simulink model "LUT_liver_pancreas_35"  (R2023b)
settings: Solver=FixedStepAuto  StartTime=0  StopTime=10.1  FixedStep=Timegap  RelTol=1e-3
model workspace (MAT data in the model file):
  T1_input = 1.34
(part 2 of 3)

== system LUT_liver_pancreas_35/If Action Subsystem6/If Action Subsystem1/If Action Subsystem6/If Action Subsystem3 ==
  In1 : Inport
  Action Port : ActionPort  ActionPortLabel=elseif( u1 >= 1.025)
  LUT 1.03RR : Lookup_n-D  NumberOfTableDimensions=1  BreakpointsForDimension1=[412.9882;555.7721;654.0253;752.1829;850.2431;948.2388;1046.193;1144.12;1242.028;1339.925;1437.812;1535.693;1633.569;1731.441;1829.31;1927.175;2025.037]  Table=[400;500;600;700;800;900;1000;1100;1200;1300;1400;1500;1600;1700;1800;1900;2000]  InternalRulePriority=Speed  RndMeth=Simplest
  Out1 : Outport
  wires:
  In1/1 -> LUT 1.03RR/1
  LUT 1.03RR/1 -> Out1/1

== system LUT_liver_pancreas_35/If Action Subsystem6/If Action Subsystem1/If Action Subsystem6/If Action Subsystem4 ==
  In1 : Inport
  Action Port : ActionPort  ActionPortLabel=elseif( u1 >= 1.035)
  LUT 1.04RR : Lookup_n-D  NumberOfTableDimensions=1  BreakpointsForDimension1=[412.8283;555.4024;653.5047;751.5005;849.3924;947.2154;1044.994;1142.743;1240.473;1338.189;1435.895;1533.595;1631.289;1728.979;1826.665;1924.348;2022.027]  Table=[400;500;600;700;800;900;1000;1100;1200;1300;1400;1500;1600;1700;1800;1900;2000]  InternalRulePriority=Speed  RndMeth=Simplest
  Out1 : Outport
  wires:
  In1/1 -> LUT 1.04RR/1
  LUT 1.04RR/1 -> Out1/1

== system LUT_liver_pancreas_35/If Action Subsystem6/If Action Subsystem1/If Action Subsystem6/If Action Subsystem5 ==
  In1 : Inport
  Action Port : ActionPort  ActionPortLabel=elseif( u1 >= 1.055)
  LUT 1.06RR : Lookup_n-D  NumberOfTableDimensions=1  BreakpointsForDimension1=[412.5162;554.689;652.5019;750.1865;847.7536;945.2432;1042.683;1140.089;1237.472;1334.84;1432.196;1529.544;1626.886;1724.223;1821.556;1918.886;2016.211]  Table=[400;500;600;700;800;900;1000;1100;1200;1300;1400;1500;1600;1700;1800;1900;2000]  InternalRulePriority=Speed  RndMeth=Simplest
  Out1 : Outport
  wires:
  In1/1 -> LUT 1.06RR/1
  LUT 1.06RR/1 -> Out1/1

== system LUT_liver_pancreas_35/If Action Subsystem6/If Action Subsystem1/If Action Subsystem6/If Action Subsystem6 ==
  In1 : Inport
  Action Port : ActionPort  ActionPortLabel=elseif( u1 >= 1.045)
  LUT 1.05RR : Lookup_n-D  NumberOfTableDimensions=1  BreakpointsForDimension1=[412.671;555.0414;652.997;750.8352;848.5627;946.2171;1043.824;1141.4;1238.955;1336.494;1434.024;1531.546;1629.062;1726.574;1824.081;1921.586;2019.086]  Table=[400;500;600;700;800;900;1000;1100;1200;1300;1400;1500;1600;1700;1800;1900;2000]  InternalRulePriority=Speed  RndMeth=Simplest
  Out1 : Outport
  wires:
  In1/1 -> LUT 1.05RR/1
  LUT 1.05RR/1 -> Out1/1

== system LUT_liver_pancreas_35/If Action Subsystem6/If Action Subsystem1/If Action Subsystem6/If Action Subsystem7 ==
  In1 : Inport
  Action Port : ActionPort  ActionPortLabel=elseif( u1 >= 1.065)
  LUT 1.07RR : Lookup_n-D  NumberOfTableDimensions=1  BreakpointsForDimension1=[412.364;554.3449;652.019;749.5538;846.9643;944.293;1041.568;1138.808;1236.024;1333.224;1430.411;1527.589;1624.76;1721.926;1819.088;1916.246;2013.4]  Table=[400;500;600;700;800;900;1000;1100;1200;1300;1400;1500;1600;1700;1800;1900;2000]  InternalRulePriority=Speed  RndMeth=Simplest
  Out1 : Outport
  wires:
  In1/1 -> LUT 1.07RR/1
  LUT 1.07RR/1 -> Out1/1

== system LUT_liver_pancreas_35/If Action Subsystem6/If Action Subsystem1/If Action Subsystem6/If Action Subsystem8 ==
  In1 : Inport
  Action Port : ActionPort  ActionPortLabel=elseif(u1 >= 1.075)
  LUT 1.08RR : Lookup_n-D  NumberOfTableDimensions=1  BreakpointsForDimension1=[412.2141;554.0089;651.5479;748.9366;846.1942;943.3656;1040.481;1137.558;1234.611;1331.645;1428.666;1525.678;1622.682;1719.681;1816.676;1913.666;2010.652]  Table=[400;500;600;700;800;900;1000;1100;1200;1300;1400;1500;1600;1700;1800;1900;2000]  InternalRulePriority=Speed  RndMeth=Simplest
  Out1 : Outport
  wires:
  In1/1 -> LUT 1.08RR/1
  LUT 1.08RR/1 -> Out1/1

== system LUT_liver_pancreas_35/If Action Subsystem6/If Action Subsystem1/If Action Subsystem6/If Action Subsystem9 ==
  In1 : Inport
  Action Port : ActionPort  ActionPortLabel=if(u1 >= 1.085)
  LUT 1.09RR : Lookup_n-D  NumberOfTableDimensions=1  BreakpointsForDimension1=[412.0667;553.6807;651.0883;748.3345;845.4429;942.4605;1039.419;1136.338;1233.23;1330.102;1426.961;1523.81;1620.651;1717.486;1814.317;1911.142;2007.964]  Table=[400;500;600;700;800;900;1000;1100;1200;1300;1400;1500;1600;1700;1800;1900;2000]  InternalRulePriority=Speed  RndMeth=Simplest
  Out1 : Outport
  wires:
  In1/1 -> LUT 1.09RR/1
  LUT 1.09RR/1 -> Out1/1

== system LUT_liver_pancreas_35/If Action Subsystem6/If Action Subsystem1/If Action Subsystem7/If Action Subsystem1 ==
  In1 : Inport
  Action Port : ActionPort  ActionPortLabel=elseif( u1 >= 1.215)
  LUT 1.22RR : Lookup_n-D  NumberOfTableDimensions=1  BreakpointsForDimension1=[410.344;550.0322;646.0176;741.6977;837.1488;932.4494;1027.65;1122.782;1217.866;1312.916;1407.94;1502.945;1597.935;1692.914;1787.883;1882.845;1977.801]  Table=[400;500;600;700;800;900;1000;1100;1200;1300;1400;1500;1600;1700;1800;1900;2000]  InternalRulePriority=Speed  RndMeth=Simplest
  Out1 : Outport
  wires:
  In1/1 -> LUT 1.22RR/1
  LUT 1.22RR/1 -> Out1/1

== system LUT_liver_pancreas_35/If Action Subsystem6/If Action Subsystem1/If Action Subsystem7/If Action Subsystem10 ==
  In1 : Inport
  Action Port : ActionPort  ActionPortLabel=elseif( u1 >= 1.205)
  LUT 1.21RR : Lookup_n-D  NumberOfTableDimensions=1  BreakpointsForDimension1=[410.4648;550.2769;646.3551;742.1389;837.701;933.1173;1028.437;1123.69;1218.897;1314.071;1409.22;1504.351;1599.467;1694.573;1789.67;1884.759;1979.843]  Table=[400;500;600;700;800;900;1000;1100;1200;1300;1400;1500;1600;1700;1800;1900;2000]  InternalRulePriority=Speed  RndMeth=Simplest
  Out1 : Outport
  wires:
  In1/1 -> LUT 1.21RR/1
  LUT 1.21RR/1 -> Out1/1

== system LUT_liver_pancreas_35/If Action Subsystem6/If Action Subsystem1/If Action Subsystem7/If Action Subsystem2 ==
  In1 : Inport
  Action Port : ActionPort  ActionPortLabel=else
  LUT 1.20RR : Lookup_n-D  NumberOfTableDimensions=1  BreakpointsForDimension1=[410.5875;550.527;646.7004;742.5906;838.2661;933.8005;1029.241;1124.618;1219.951;1315.251;1410.528;1505.787;1601.032;1696.267;1791.493;1886.713;1981.926]  Table=[400;500;600;700;800;900;1000;1100;1200;1300;1400;1500;1600;1700;1800;1900;2000]  InternalRulePriority=Speed  RndMeth=Simplest
  Out1 : Outport
  wires:
  In1/1 -> LUT 1.20RR/1
  LUT 1.20RR/1 -> Out1/1

== system LUT_liver_pancreas_35/If Action Subsystem6/If Action Subsystem1/If Action Subsystem7/If Action Subsystem3 ==
  In1 : Inport
  Action Port : ActionPort  ActionPortLabel=elseif( u1 >= 1.225)
  LUT 1.23RR : Lookup_n-D  NumberOfTableDimensions=1  BreakpointsForDimension1=[410.2248;549.7928;645.6879;741.2665;836.6092;931.7964;1026.88;1121.894;1216.857;1311.785;1406.686;1501.568;1596.434;1691.288;1786.133;1880.969;1975.8]  Table=[400;500;600;700;800;900;1000;1100;1200;1300;1400;1500;1600;1700;1800;1900;2000]  InternalRulePriority=Speed  RndMeth=Simplest
  Out1 : Outport
  wires:
  In1/1 -> LUT 1.23RR/1
  LUT 1.23RR/1 -> Out1/1

== system LUT_liver_pancreas_35/If Action Subsystem6/If Action Subsystem1/If Action Subsystem7/If Action Subsystem4 ==
  In1 : Inport
  Action Port : ActionPort  ActionPortLabel=elseif( u1 >= 1.235)
  LUT 1.24RR : Lookup_n-D  NumberOfTableDimensions=1  BreakpointsForDimension1=[410.1074;549.5585;645.3656;740.8452;836.0817;931.158;1026.128;1121.024;1215.87;1310.678;1405.459;1500.219;1594.963;1689.695;1784.417;1879.131;1973.838]  Table=[400;500;600;700;800;900;1000;1100;1200;1300;1400;1500;1600;1700;1800;1900;2000]  InternalRulePriority=Speed  RndMeth=Simplest
  Out1 : Outport
  wires:
  In1/1 -> LUT 1.24RR/1
  LUT 1.24RR/1 -> Out1/1

== system LUT_liver_pancreas_35/If Action Subsystem6/If Action Subsystem1/If Action Subsystem7/If Action Subsystem5 ==
  In1 : Inport
  Action Port : ActionPort  ActionPortLabel=elseif( u1 >= 1.255)
  LUT 1.26RR : Lookup_n-D  NumberOfTableDimensions=1  BreakpointsForDimension1=[409.8775;549.1047;644.7426;740.031;835.062;929.9232;1024.671;1119.341;1213.957;1308.533;1403.079;1497.603;1592.111;1686.605;1781.088;1875.562;1970.03]  Table=[400;500;600;700;800;900;1000;1100;1200;1300;1400;1500;1600;1700;1800;1900;2000]  InternalRulePriority=Speed  RndMeth=Simplest
  Out1 : Outport
  wires:
  In1/1 -> LUT 1.26RR/1
  LUT 1.26RR/1 -> Out1/1

== system LUT_liver_pancreas_35/If Action Subsystem6/If Action Subsystem1/If Action Subsystem7/If Action Subsystem6 ==
  In1 : Inport
  Action Port : ActionPort  ActionPortLabel=elseif( u1 >= 1.245)
  LUT 1.25RR : Lookup_n-D  NumberOfTableDimensions=1  BreakpointsForDimension1=[409.9916;549.3292;645.0505;740.4334;835.566;930.5337;1025.391;1120.174;1214.903;1309.594;1404.257;1498.898;1593.522;1688.134;1782.736;1877.329;1971.915]  Table=[400;500;600;700;800;900;1000;1100;1200;1300;1400;1500;1600;1700;1800;1900;2000]  InternalRulePriority=Speed  RndMeth=Simplest
  Out1 : Outport
  wires:
  In1/1 -> LUT 1.25RR/1
  LUT 1.25RR/1 -> Out1/1

== system LUT_liver_pancreas_35/If Action Subsystem6/If Action Subsystem1/If Action Subsystem7/If Action Subsystem7 ==
  In1 : Inport
  Action Port : ActionPort  ActionPortLabel=elseif( u1 >= 1.265)
  LUT 1.27RR : Lookup_n-D  NumberOfTableDimensions=1  BreakpointsForDimension1=[409.765;548.8849;644.4415;739.6376;834.5691;929.3261;1023.966;1118.527;1213.03;1307.493;1401.926;1496.335;1590.727;1685.105;1779.472;1873.83;1968.181]  Table=[400;500;600;700;800;900;1000;1100;1200;1300;1400;1500;1600;1700;1800;1900;2000]  InternalRulePriority=Speed  RndMeth=Simplest
  Out1 : Outport
  wires:
  In1/1 -> LUT 1.27RR/1
  LUT 1.27RR/1 -> Out1/1

== system LUT_liver_pancreas_35/If Action Subsystem6/If Action Subsystem1/If Action Subsystem7/If Action Subsystem8 ==
  In1 : Inport
  Action Port : ActionPort  ActionPortLabel=elseif(u1 >= 1.275)
  LUT 1.28RR : Lookup_n-D  NumberOfTableDimensions=1  BreakpointsForDimension1=[409.654;548.6697;644.1471;739.2531;834.0873;928.7421;1023.277;1117.729;1212.123;1306.475;1400.796;1495.093;1589.371;1683.635;1777.888;1872.132;1966.368]  Table=[400;500;600;700;800;900;1000;1100;1200;1300;1400;1500;1600;1700;1800;1900;2000]  InternalRulePriority=Speed  RndMeth=Simplest
  Out1 : Outport
  wires:
  In1/1 -> LUT 1.28RR/1
  LUT 1.28RR/1 -> Out1/1

== system LUT_liver_pancreas_35/If Action Subsystem6/If Action Subsystem1/If Action Subsystem7/If Action Subsystem9 ==
  In1 : Inport
  Action Port : ActionPort  ActionPortLabel=if(u1 >= 1.285)
  LUT 1.29RR : Lookup_n-D  NumberOfTableDimensions=1  BreakpointsForDimension1=[409.5446;548.459;643.8592;738.8772;833.6161;928.1708;1022.602;1116.949;1211.235;1305.478;1399.689;1493.875;1588.042;1682.195;1776.335;1870.466;1964.589]  Table=[400;500;600;700;800;900;1000;1100;1200;1300;1400;1500;1600;1700;1800;1900;2000]  InternalRulePriority=Speed  RndMeth=Simplest
  Out1 : Outport
  wires:
  In1/1 -> LUT 1.29RR/1
  LUT 1.29RR/1 -> Out1/1

== system LUT_liver_pancreas_35/If Action Subsystem6/If Action Subsystem1/If Action Subsystem8/If Action Subsystem1 ==
  In1 : Inport
  Action Port : ActionPort  ActionPortLabel=elseif( u1 >= 1.315)
  LUT 1.32RR : Lookup_n-D  NumberOfTableDimensions=1  BreakpointsForDimension1=[409.2254;547.8525;643.0331;737.7988;832.2639;926.5301;1020.663;1114.703;1208.679;1302.606;1396.499;1490.364;1584.209;1678.038;1771.853;1865.658;1959.455]  Table=[400;500;600;700;800;900;1000;1100;1200;1300;1400;1500;1600;1700;1800;1900;2000]  InternalRulePriority=Speed  RndMeth=Simplest
  Out1 : Outport
  wires:
  In1/1 -> LUT 1.32RR/1
  LUT 1.32RR/1 -> Out1/1

== system LUT_liver_pancreas_35/If Action Subsystem6/If Action Subsystem1/If Action Subsystem8/If Action Subsystem10 ==
  In1 : Inport
  Action Port : ActionPort  ActionPortLabel=elseif( u1 >= 1.305)
  LUT 1.31RR : Lookup_n-D  NumberOfTableDimensions=1  BreakpointsForDimension1=[409.3303;548.0505;643.3024;738.1503;832.7047;927.0651;1021.295;1115.436;1209.513;1303.544;1397.541;1491.511;1585.462;1679.396;1773.318;1867.23;1961.134]  Table=[400;500;600;700;800;900;1000;1100;1200;1300;1400;1500;1600;1700;1800;1900;2000]  InternalRulePriority=Speed  RndMeth=Simplest
  Out1 : Outport
  wires:
  In1/1 -> LUT 1.31RR/1
  LUT 1.31RR/1 -> Out1/1

== system LUT_liver_pancreas_35/If Action Subsystem6/If Action Subsystem1/If Action Subsystem8/If Action Subsystem2 ==
  In1 : Inport
  Action Port : ActionPort  ActionPortLabel=else
  LUT 1.30RR : Lookup_n-D  NumberOfTableDimensions=1  BreakpointsForDimension1=[409.4368;548.2526;643.5777;738.5096;833.1553;927.6119;1021.942;1116.184;1210.365;1304.501;1398.604;1492.681;1586.739;1680.782;1774.812;1868.833;1962.845]  Table=[400;500;600;700;800;900;1000;1100;1200;1300;1400;1500;1600;1700;1800;1900;2000]  InternalRulePriority=Speed  RndMeth=Simplest
  Out1 : Outport
  wires:
  In1/1 -> LUT 1.30RR/1
  LUT 1.30RR/1 -> Out1/1

== system LUT_liver_pancreas_35/If Action Subsystem6/If Action Subsystem1/If Action Subsystem8/If Action Subsystem3 ==
  In1 : Inport
  Action Port : ActionPort  ActionPortLabel=elseif( u1 >= 1.325)
  LUT 1.33RR : Lookup_n-D  NumberOfTableDimensions=1  BreakpointsForDimension1=[409.1218;547.6585;642.7698;737.4552;831.8328;926.0066;1020.044;1113.986;1207.861;1301.687;1395.478;1489.24;1582.981;1676.705;1770.416;1864.116;1957.807]  Table=[400;500;600;700;800;900;1000;1100;1200;1300;1400;1500;1600;1700;1800;1900;2000]  InternalRulePriority=Speed  RndMeth=Simplest
  Out1 : Outport
  wires:
  In1/1 -> LUT 1.33RR/1
  LUT 1.33RR/1 -> Out1/1

== system LUT_liver_pancreas_35/If Action Subsystem6/If Action Subsystem1/If Action Subsystem8/If Action Subsystem4 ==
  In1 : Inport
  Action Port : ActionPort  ActionPortLabel=elseif( u1 >= 1.335)
  LUT 1.34RR : Lookup_n-D  NumberOfTableDimensions=1  BreakpointsForDimension1=[409.0197;547.4685;642.5121;737.1191;831.4111;925.4944;1019.437;1113.283;1207.06;1300.787;1394.476;1488.137;1581.776;1675.398;1769.006;1862.603;1956.19]  Table=[400;500;600;700;800;900;1000;1100;1200;1300;1400;1500;1600;1700;1800;1900;2000]  InternalRulePriority=Speed  RndMeth=Simplest
  Out1 : Outport
  wires:
  In1/1 -> LUT 1.34RR/1
  LUT 1.34RR/1 -> Out1/1

== system LUT_liver_pancreas_35/If Action Subsystem6/If Action Subsystem1/If Action Subsystem8/If Action Subsystem5 ==
  In1 : Inport
  Action Port : ActionPort  ActionPortLabel=elseif( u1 >= 1.355)
  LUT 1.36RR : Lookup_n-D  NumberOfTableDimensions=1  BreakpointsForDimension1=[408.8194;547.0998;642.0134;736.4689;830.595;924.5024;1018.263;1111.921;1205.507;1299.039;1392.533;1485.996;1579.436;1672.858;1766.265;1859.66;1953.046]  Table=[400;500;600;700;800;900;1000;1100;1200;1300;1400;1500;1600;1700;1800;1900;2000]  InternalRulePriority=Speed  RndMeth=Simplest
  Out1 : Outport
  wires:
  In1/1 -> LUT 1.36RR/1
  LUT 1.36RR/1 -> Out1/1

== system LUT_liver_pancreas_35/If Action Subsystem6/If Action Subsystem1/If Action Subsystem8/If Action Subsystem6 ==
  In1 : Inport
  Action Port : ActionPort  ActionPortLabel=elseif( u1 >= 1.345)
  LUT 1.35RR : Lookup_n-D  NumberOfTableDimensions=1  BreakpointsForDimension1=[408.9189;547.2823;642.26;736.7904;830.9986;924.9931;1018.844;1112.595;1206.276;1299.904;1393.495;1487.056;1580.595;1674.116;1767.623;1861.118;1954.603]  Table=[400;500;600;700;800;900;1000;1100;1200;1300;1400;1500;1600;1700;1800;1900;2000]  InternalRulePriority=Speed  RndMeth=Simplest
  Out1 : Outport
  wires:
  In1/1 -> LUT 1.35RR/1
  LUT 1.35RR/1 -> Out1/1

== system LUT_liver_pancreas_35/If Action Subsystem6/If Action Subsystem1/If Action Subsystem8/If Action Subsystem7 ==
  In1 : Inport
  Action Port : ActionPort  ActionPortLabel=elseif( u1 >= 1.365)
  LUT 1.37RR : Lookup_n-D  NumberOfTableDimensions=1  BreakpointsForDimension1=[408.7213;546.921;641.7721;736.1544;830.2001;924.0222;1017.694;1111.261;1204.753;1298.192;1391.589;1484.956;1578.299;1671.624;1764.933;1858.23;1951.517]  Table=[400;500;600;700;800;900;1000;1100;1200;1300;1400;1500;1600;1700;1800;1900;2000]  InternalRulePriority=Speed  RndMeth=Simplest
  Out1 : Outport
  wires:
  In1/1 -> LUT 1.37RR/1
  LUT 1.37RR/1 -> Out1/1

== system LUT_liver_pancreas_35/If Action Subsystem6/If Action Subsystem1/If Action Subsystem8/If Action Subsystem8 ==
  In1 : Inport
  Action Port : ActionPort  ActionPortLabel=elseif(u1 >= 1.375)
  LUT 1.38RR : Lookup_n-D  NumberOfTableDimensions=1  BreakpointsForDimension1=[408.6244;546.7457;641.5359;735.8468;829.8137;923.5522;1017.136;1110.614;1204.015;1297.36;1390.664;1483.937;1577.184;1670.413;1763.625;1856.826;1950.016]  Table=[400;500;600;700;800;900;1000;1100;1200;1300;1400;1500;1600;1700;1800;1900;2000]  InternalRulePriority=Speed  RndMeth=Simplest
  Out1 : Outport
  wires:
  In1/1 -> LUT 1.38RR/1
  LUT 1.38RR/1 -> Out1/1

== system LUT_liver_pancreas_35/If Action Subsystem6/If Action Subsystem1/If Action Subsystem8/If Action Subsystem9 ==
  In1 : Inport
  Action Port : ActionPort  ActionPortLabel=if(u1 >= 1.385)
  LUT 1.39RR : Lookup_n-D  NumberOfTableDimensions=1  BreakpointsForDimension1=[408.5288;546.5738;641.3049;735.5459;829.4357;923.0921;1016.591;1109.98;1203.291;1296.545;1389.757;1482.936;1576.09;1669.224;1762.342;1855.447;1948.542]  Table=[400;500;600;700;800;900;1000;1100;1200;1300;1400;1500;1600;1700;1800;1900;2000]  InternalRulePriority=Speed  RndMeth=Simplest
  Out1 : Outport
  wires:
  In1/1 -> LUT 1.39RR/1
  LUT 1.39RR/1 -> Out1/1

== system LUT_liver_pancreas_35/If Action Subsystem6/If Action Subsystem1/If Action Subsystem9/If Action Subsystem1 ==
  In1 : Inport
  Action Port : ActionPort  ActionPortLabel=elseif( u1 >= 1.415)
  LUT 1.42RR : Lookup_n-D  NumberOfTableDimensions=1  BreakpointsForDimension1=[408.2493167;546.0782587;640.6407138;734.6814994;828.3494623;921.7690503;1015.020415;1108.154745;1201.205449;1294.194915;1387.138542;1480.047175;1572.92862;1665.788602;1758.631391;1851.460216;1944.277551]  Table=[400;500;600;700;800;900;1000;1100;1200;1300;1400;1500;1600;1700;1800;1900;2000]  InternalRulePriority=Speed  RndMeth=Simplest
  Out1 : Outport
  wires:
  In1/1 -> LUT 1.42RR/1
  LUT 1.42RR/1 -> Out1/1

== system LUT_liver_pancreas_35/If Action Subsystem6/If Action Subsystem1/If Action Subsystem9/If Action Subsystem10 ==
  In1 : Inport
  Action Port : ActionPort  ActionPortLabel=elseif( u1 >= 1.405)
  LUT 1.41RR : Lookup_n-D  NumberOfTableDimensions=1  BreakpointsForDimension1=[408.3412832;546.2402113;640.8573639;734.9633581;828.7037439;922.2007473;1015.533048;1108.750853;1201.886902;1294.96312;1387.994576;1480.99188;1573.962659;1666.912507;1759.845592;1852.765065;1945.673336]  Table=[400;500;600;700;800;900;1000;1100;1200;1300;1400;1500;1600;1700;1800;1900;2000]  InternalRulePriority=Speed  RndMeth=Simplest
  Out1 : Outport
  wires:
  In1/1 -> LUT 1.41RR/1
  LUT 1.41RR/1 -> Out1/1

== system LUT_liver_pancreas_35/If Action Subsystem6/If Action Subsystem1/If Action Subsystem9/If Action Subsystem2 ==
  In1 : Inport
  Action Port : ActionPort  ActionPortLabel=else
  LUT 1.40RR : Lookup_n-D  NumberOfTableDimensions=1  BreakpointsForDimension1=[408.4344;546.4054;641.0787;735.2514;829.0658;922.6417;1016.056;1109.359;1202.582;1295.747;1388.867;1481.955;1575.016;1668.057;1761.082;1854.094;1947.095]  Table=[400;500;600;700;800;900;1000;1100;1200;1300;1400;1500;1600;1700;1800;1900;2000]  InternalRulePriority=Speed  RndMeth=Simplest
  Out1 : Outport
  wires:
  In1/1 -> LUT 1.40RR/1
  LUT 1.40RR/1 -> Out1/1

== system LUT_liver_pancreas_35/If Action Subsystem6/If Action Subsystem1/If Action Subsystem9/If Action Subsystem3 ==
  In1 : Inport
  Action Port : ActionPort  ActionPortLabel=elseif( u1 >= 1.425)
  LUT 1.43RR : Lookup_n-D  NumberOfTableDimensions=1  BreakpointsForDimension1=[408.1585;545.9194;640.4286;734.4057;828.0027;921.3464;1014.518;1107.571;1200.537;1293.442;1386.299;1479.12;1571.914;1664.685;1757.439;1850.179;1942.907]  Table=[400;500;600;700;800;900;1000;1100;1200;1300;1400;1500;1600;1700;1800;1900;2000]  InternalRulePriority=Speed  RndMeth=Simplest
  Out1 : Outport
  wires:
  In1/1 -> LUT 1.43RR/1
  LUT 1.43RR/1 -> Out1/1

== system LUT_liver_pancreas_35/If Action Subsystem6/If Action Subsystem1/If Action Subsystem9/If Action Subsystem4 ==
  In1 : Inport
  Action Port : ActionPort  ActionPortLabel=elseif( u1 >= 1.435)
  LUT 1.44RR : Lookup_n-D  NumberOfTableDimensions=1  BreakpointsForDimension1=[408.0689;545.7637;640.221;734.1358;827.6634;920.9325;1014.026;1106.998;1199.882;1292.703;1385.475;1478.211;1570.918;1663.602;1756.269;1848.92;1941.56]  Table=[400;500;600;700;800;900;1000;1100;1200;1300;1400;1500;1600;1700;1800;1900;2000]  InternalRulePriority=Speed  RndMeth=Simplest
  Out1 : Outport
  wires:
  In1/1 -> LUT 1.44RR/1
  LUT 1.44RR/1 -> Out1/1

== system LUT_liver_pancreas_35/If Action Subsystem6/If Action Subsystem1/If Action Subsystem9/If Action Subsystem5 ==
  In1 : Inport
  Action Port : ActionPort  ActionPortLabel=elseif( u1 >= 1.455)
  LUT 1.46RR : Lookup_n-D  NumberOfTableDimensions=1  BreakpointsForDimension1=[407.8929;545.4611;639.8188;733.6133;827.0061;920.1305;1013.073;1105.887;1198.611;1291.267;1383.874;1476.442;1568.98;1661.494;1753.99;1846.47;1938.937]  Table=[400;500;600;700;800;900;1000;1100;1200;1300;1400;1500;1600;1700;1800;1900;2000]  InternalRulePriority=Speed  RndMeth=Simplest
  Out1 : Outport
  wires:
  In1/1 -> LUT 1.46RR/1
  LUT 1.46RR/1 -> Out1/1

== system LUT_liver_pancreas_35/If Action Subsystem6/If Action Subsystem1/If Action Subsystem9/If Action Subsystem6 ==
  In1 : Inport
  Action Port : ActionPort  ActionPortLabel=elseif( u1 >= 1.445)
  LUT 1.45RR : Lookup_n-D  NumberOfTableDimensions=1  BreakpointsForDimension1=[407.9803;545.6109;640.0178;733.8717;827.3312;920.5273;1013.545;1106.437;1199.24;1291.978;1384.667;1477.318;1569.94;1662.539;1755.119;1847.684;1940.237]  Table=[400;500;600;700;800;900;1000;1100;1200;1300;1400;1500;1600;1700;1800;1900;2000]  InternalRulePriority=Speed  RndMeth=Simplest
  Out1 : Outport
  wires:
  In1/1 -> LUT 1.45RR/1
  LUT 1.45RR/1 -> Out1/1

== system LUT_liver_pancreas_35/If Action Subsystem6/If Action Subsystem1/If Action Subsystem9/If Action Subsystem7 ==
  In1 : Inport
  Action Port : ActionPort  ActionPortLabel=elseif( u1 >= 1.465)
  LUT 1.47RR : Lookup_n-D  NumberOfTableDimensions=1  BreakpointsForDimension1=[407.8066;545.3141;639.624;733.3604;826.6879;919.7419;1012.61;1105.348;1197.993;1290.57;1383.096;1475.582;1568.037;1660.469;1752.881;1845.277;1937.66]  Table=[400;500;600;700;800;900;1000;1100;1200;1300;1400;1500;1600;1700;1800;1900;2000]  InternalRulePriority=Speed  RndMeth=Simplest
  Out1 : Outport
  wires:
  In1/1 -> LUT 1.47RR/1
  LUT 1.47RR/1 -> Out1/1

== system LUT_liver_pancreas_35/If Action Subsystem6/If Action Subsystem1/If Action Subsystem9/If Action Subsystem8 ==
  In1 : Inport
  Action Port : ActionPort  ActionPortLabel=elseif(u1 >= 1.475)
  LUT 1.48RR : Lookup_n-D  NumberOfTableDimensions=1  BreakpointsForDimension1=[407.7213;545.1698;639.4333;733.1128;826.3764;919.3614;1012.157;1104.82;1197.388;1289.886;1382.332;1474.738;1567.112;1659.462;1751.792;1844.105;1936.406]  Table=[400;500;600;700;800;900;1000;1100;1200;1300;1400;1500;1600;1700;1800;1900;2000]  InternalRulePriority=Speed  RndMeth=Simplest
  Out1 : Outport
  wires:
  In1/1 -> LUT 1.48RR/1
  LUT 1.48RR/1 -> Out1/1

== system LUT_liver_pancreas_35/If Action Subsystem6/If Action Subsystem1/If Action Subsystem9/If Action Subsystem9 ==
  In1 : Inport
  Action Port : ActionPort  ActionPortLabel=if(u1 >= 1.485)
  LUT 1.49RR : Lookup_n-D  NumberOfTableDimensions=1  BreakpointsForDimension1=[407.637;545.0283;639.2465;732.8705;826.0714;918.9888;1011.713;1104.302;1196.794;1289.215;1381.583;1473.909;1566.203;1658.473;1750.721;1842.954;1935.173]  Table=[400;500;600;700;800;900;1000;1100;1200;1300;1400;1500;1600;1700;1800;1900;2000]  InternalRulePriority=Speed  RndMeth=Simplest
  Out1 : Outport
  wires:
  In1/1 -> LUT 1.49RR/1
  LUT 1.49RR/1 -> Out1/1

== system LUT_liver_pancreas_35/If Action Subsystem6/If Action Subsystem2/If Action Subsystem5/If Action Subsystem1 ==
  In1 : Inport
  Action Port : ActionPort  ActionPortLabel=elseif( u1 >= 1.615)
  LUT 1.62RR : Lookup_n-D  NumberOfTableDimensions=1  BreakpointsForDimension1=[406.6287;543.4093;637.1404;730.1493;822.6427;914.7867;1006.69;1098.424;1190.035;1281.556;1373.008;1464.407;1555.765;1647.09;1738.389;1829.666;1920.925]  Table=[400;500;600;700;800;900;1000;1100;1200;1300;1400;1500;1600;1700;1800;1900;2000]  InternalRulePriority=Speed  RndMeth=Simplest
  Out1 : Outport
  wires:
  In1/1 -> LUT 1.62RR/1
  LUT 1.62RR/1 -> Out1/1

== system LUT_liver_pancreas_35/If Action Subsystem6/If Action Subsystem2/If Action Subsystem5/If Action Subsystem10 ==
  In1 : Inport
  Action Port : ActionPort  ActionPortLabel=elseif( u1>= 1.605)
  LUT 1.61RR : Lookup_n-D  NumberOfTableDimensions=1  BreakpointsForDimension1=[406.701;543.5206;637.2832;730.333;822.8743;915.0714;1007.032;1098.825;1190.498;1282.081;1373.597;1465.061;1556.485;1647.877;1739.242;1830.587;1921.914]  Table=[400;500;600;700;800;900;1000;1100;1200;1300;1400;1500;1600;1700;1800;1900;2000]  InternalRulePriority=Speed  RndMeth=Simplest
  Out1 : Outport
  wires:
  In1/1 -> LUT 1.61RR/1
  LUT 1.61RR/1 -> Out1/1

== system LUT_liver_pancreas_35/If Action Subsystem6/If Action Subsystem2/If Action Subsystem5/If Action Subsystem2 ==
  In1 : Inport
  Action Port : ActionPort  ActionPortLabel=else
  LUT 1.60RR : Lookup_n-D  NumberOfTableDimensions=1  BreakpointsForDimension1=[406.7741;543.634;637.4289;730.5206;823.1109;915.362;1007.38;1099.234;1190.969;1282.616;1374.197;1465.728;1557.218;1648.677;1740.111;1831.523;1922.919]  Table=[400;500;600;700;800;900;1000;1100;1200;1300;1400;1500;1600;1700;1800;1900;2000]  InternalRulePriority=Speed  RndMeth=Simplest
  Out1 : Outport
  wires:
  In1/1 -> LUT 1.60RR/1
  LUT 1.60RR/1 -> Out1/1

== system LUT_liver_pancreas_35/If Action Subsystem6/If Action Subsystem2/If Action Subsystem5/If Action Subsystem3 ==
  In1 : Inport
  Action Port : ActionPort  ActionPortLabel=elseif( u1 >= 1.625)
  LUT 1.63RR : Lookup_n-D  NumberOfTableDimensions=1  BreakpointsForDimension1=[406.5573;543.2999;637.0006;729.9695;822.4159;914.5078;1006.356;1098.031;1189.582;1281.04;1372.429;1463.764;1555.057;1646.317;1737.549;1828.76;1919.953]  Table=[400;500;600;700;800;900;1000;1100;1200;1300;1400;1500;1600;1700;1800;1900;2000]  InternalRulePriority=Speed  RndMeth=Simplest
  Out1 : Outport
  wires:
  In1/1 -> LUT 1.63RR/1
  LUT 1.63RR/1 -> Out1/1

== system LUT_liver_pancreas_35/If Action Subsystem6/If Action Subsystem2/If Action Subsystem5/If Action Subsystem4 ==
  In1 : Inport
  Action Port : ActionPort  ActionPortLabel=elseif( u1 >= 1.635)
  LUT 1.64RR : Lookup_n-D  NumberOfTableDimensions=1  BreakpointsForDimension1=[406.4867;543.1924;636.8635;729.7934;822.1938;914.2347;1006.028;1097.646;1189.137;1280.534;1371.861;1463.132;1554.361;1645.556;1736.724;1827.869;1918.997]  Table=[400;500;600;700;800;900;1000;1100;1200;1300;1400;1500;1600;1700;1800;1900;2000]  InternalRulePriority=Speed  RndMeth=Simplest
  Out1 : Outport
  wires:
  In1/1 -> LUT 1.64RR/1
  LUT 1.64RR/1 -> Out1/1

== system LUT_liver_pancreas_35/If Action Subsystem6/If Action Subsystem2/If Action Subsystem5/If Action Subsystem5 ==
  In1 : Inport
  Action Port : ActionPort  ActionPortLabel=elseif( u1 >= 1.655)
  LUT 1.66RR : Lookup_n-D  NumberOfTableDimensions=1  BreakpointsForDimension1=[406.3478;542.983;636.5976;729.4522;821.7633;913.7049;1005.391;1096.897;1188.272;1279.55;1370.754;1461.902;1553.006;1644.075;1735.115;1826.132;1917.13]  Table=[400;500;600;700;800;900;1000;1100;1200;1300;1400;1500;1600;1700;1800;1900;2000]  InternalRulePriority=Speed  RndMeth=Simplest
  Out1 : Outport
  wires:
  In1/1 -> LUT 1.66RR/1
  LUT 1.66RR/1 -> Out1/1

== system LUT_liver_pancreas_35/If Action Subsystem6/If Action Subsystem2/If Action Subsystem5/If Action Subsystem6 ==
  In1 : Inport
  Action Port : ActionPort  ActionPortLabel=elseif( u1 >= 1.645)
  LUT 1.65RR : Lookup_n-D  NumberOfTableDimensions=1  BreakpointsForDimension1=[406.4168;543.0868;636.7292;729.621;821.9763;913.967;1005.706;1097.268;1188.7;1280.037;1371.302;1462.512;1553.678;1644.809;1735.913;1826.994;1918.056]  Table=[400;500;600;700;800;900;1000;1100;1200;1300;1400;1500;1600;1700;1800;1900;2000]  InternalRulePriority=Speed  RndMeth=Simplest
  Out1 : Outport
  wires:
  In1/1 -> LUT 1.65RR/1
  LUT 1.65RR/1 -> Out1/1

== system LUT_liver_pancreas_35/If Action Subsystem6/If Action Subsystem2/If Action Subsystem5/If Action Subsystem7 ==
  In1 : Inport
  Action Port : ActionPort  ActionPortLabel=elseif( u1 >= 1.665)
  LUT 1.67RR : Lookup_n-D  NumberOfTableDimensions=1  BreakpointsForDimension1=[406.2795;542.8811;636.4686;729.2869;821.5548;913.448;1005.082;1096.533;1187.851;1279.071;1370.216;1461.303;1552.346;1643.352;1734.33;1825.285;1916.22]  Table=[400;500;600;700;800;900;1000;1100;1200;1300;1400;1500;1600;1700;1800;1900;2000]  InternalRulePriority=Speed  RndMeth=Simplest
  Out1 : Outport
  wires:
  In1/1 -> LUT 1.67RR/1
  LUT 1.67RR/1 -> Out1/1

== system LUT_liver_pancreas_35/If Action Subsystem6/If Action Subsystem2/If Action Subsystem5/If Action Subsystem8 ==
  In1 : Inport
  Action Port : ActionPort  ActionPortLabel=elseif(u1 >= 1.675)
  LUT 1.68RR : Lookup_n-D  NumberOfTableDimensions=1  BreakpointsForDimension1=[406.2119;542.7809;636.3422;729.1251;821.3507;913.1965;1004.78;1096.177;1187.439;1278.601;1369.687;1460.715;1551.697;1642.643;1733.559;1824.451;1915.324]  Table=[400;500;600;700;800;900;1000;1100;1200;1300;1400;1500;1600;1700;1800;1900;2000]  InternalRulePriority=Speed  RndMeth=Simplest
  Out1 : Outport
  wires:
  In1/1 -> LUT 1.68RR/1
  LUT 1.68RR/1 -> Out1/1

== system LUT_liver_pancreas_35/If Action Subsystem6/If Action Subsystem2/If Action Subsystem5/If Action Subsystem9 ==
  In1 : Inport
  Action Port : ActionPort  ActionPortLabel=if(u1 >= 1.685)
  LUT 1.69RR : Lookup_n-D  NumberOfTableDimensions=1  BreakpointsForDimension1=[406.1451;542.6825;636.2183;728.9667;821.1508;912.95;1004.483;1095.827;1187.034;1278.139;1369.168;1460.137;1551.059;1641.945;1732.8;1823.631;1914.442]  Table=[400;500;600;700;800;900;1000;1100;1200;1300;1400;1500;1600;1700;1800;1900;2000]  InternalRulePriority=Speed  RndMeth=Simplest
  Out1 : Outport
  wires:
  In1/1 -> LUT 1.69RR/1
  LUT 1.69RR/1 -> Out1/1

== system LUT_liver_pancreas_35/If Action Subsystem6/If Action Subsystem2/If Action Subsystem6/If Action Subsystem1 ==
  In1 : Inport
  Action Port : ActionPort  ActionPortLabel=elseif( u1 >= 1.515)
  LUT 1.52RR : Lookup_n-D  NumberOfTableDimensions=1  BreakpointsForDimension1=[407.3904;544.6195;638.709;732.1741;825.1945;917.9163;1010.434;1102.809;1195.081;1287.278;1379.417;1471.513;1563.575;1655.61;1747.623;1839.618;1931.599]  Table=[400;500;600;700;800;900;1000;1100;1200;1300;1400;1500;1600;1700;1800;1900;2000]  InternalRulePriority=Speed  RndMeth=Simplest
  Out1 : Outport
  wires:
  In1/1 -> LUT 1.52RR/1
  LUT 1.52RR/1 -> Out1/1

== system LUT_liver_pancreas_35/If Action Subsystem6/If Action Subsystem2/If Action Subsystem6/If Action Subsystem10 ==
  In1 : Inport
  Action Port : ActionPort  ActionPortLabel=elseif( u1 >= 1.505)
  LUT 1.51RR : Lookup_n-D  NumberOfTableDimensions=1  BreakpointsForDimension1=[407.4716;544.7532;638.8844;732.4013;825.4806;918.2664;1010.852;1103.297;1195.641;1287.911;1380.125;1472.297;1564.435;1656.547;1748.637;1840.711;1932.77]  Table=[400;500;600;700;800;900;1000;1100;1200;1300;1400;1500;1600;1700;1800;1900;2000]  InternalRulePriority=Speed  RndMeth=Simplest
  Out1 : Outport
  wires:
  In1/1 -> LUT 1.51RR/1
  LUT 1.51RR/1 -> Out1/1

== system LUT_liver_pancreas_35/If Action Subsystem6/If Action Subsystem2/If Action Subsystem6/If Action Subsystem2 ==
  In1 : Inport
  Action Port : ActionPort  ActionPortLabel=else
  LUT 1.50RR : Lookup_n-D  NumberOfTableDimensions=1  BreakpointsForDimension1=[407.5538;544.8895;639.0635;732.6334;825.7729;918.6238;1011.278;1103.795;1196.212;1288.557;1380.847;1473.096;1565.311;1657.501;1749.67;1841.823;1933.961]  Table=[400;500;600;700;800;900;1000;1100;1200;1300;1400;1500;1600;1700;1800;1900;2000]  InternalRulePriority=Speed  RndMeth=Simplest
  Out1 : Outport
  wires:
  In1/1 -> LUT 1.50RR/1
  LUT 1.50RR/1 -> Out1/1

== system LUT_liver_pancreas_35/If Action Subsystem6/If Action Subsystem2/If Action Subsystem6/If Action Subsystem3 ==
  In1 : Inport
  Action Port : ActionPort  ActionPortLabel=elseif( u1 >= 1.525)
  LUT 1.53RR : Lookup_n-D  NumberOfTableDimensions=1  BreakpointsForDimension1=[407.3101;544.4882;638.5372;731.9517;824.9144;917.5734;1010.025;1102.331;1194.532;1286.656;1378.722;1470.743;1562.73;1654.689;1746.626;1838.545;1930.449]  Table=[400;500;600;700;800;900;1000;1100;1200;1300;1400;1500;1600;1700;1800;1900;2000]  InternalRulePriority=Speed  RndMeth=Simplest
  Out1 : Outport
  wires:
  In1/1 -> LUT 1.53RR/1
  LUT 1.53RR/1 -> Out1/1

== system LUT_liver_pancreas_35/If Action Subsystem6/If Action Subsystem2/If Action Subsystem6/If Action Subsystem4 ==
  In1 : Inport
  Action Port : ActionPort  ActionPortLabel=elseif( u1 >= 1.535)
  LUT 1.54RR : Lookup_n-D  NumberOfTableDimensions=1  BreakpointsForDimension1=[407.2308;544.3594;638.3689;731.734;824.6401;917.2375;1009.624;1101.862;1193.993;1286.046;1378.039;1469.987;1561.9;1653.784;1745.646;1837.489;1929.318]  Table=[400;500;600;700;800;900;1000;1100;1200;1300;1400;1500;1600;1700;1800;1900;2000]  InternalRulePriority=Speed  RndMeth=Simplest
  Out1 : Outport
  wires:
  In1/1 -> LUT 1.54RR/1
  LUT 1.54RR/1 -> Out1/1

== system LUT_liver_pancreas_35/If Action Subsystem6/If Action Subsystem2/If Action Subsystem6/If Action Subsystem5 ==
  In1 : Inport
  Action Port : ActionPort  ActionPortLabel=elseif( u1 >= 1.555)
  LUT 1.56RR : Lookup_n-D  NumberOfTableDimensions=1  BreakpointsForDimension1=[407.075;544.1087;638.0426;731.3122;824.1087;916.5864;1008.846;1100.951;1192.946;1284.859;1376.711;1468.516;1560.283;1652.022;1743.737;1835.432;1927.112]  Table=[400;500;600;700;800;900;1000;1100;1200;1300;1400;1500;1600;1700;1800;1900;2000]  InternalRulePriority=Speed  RndMeth=Simplest
  Out1 : Outport
  wires:
  In1/1 -> LUT 1.56RR/1
  LUT 1.56RR/1 -> Out1/1

== system LUT_liver_pancreas_35/If Action Subsystem6/If Action Subsystem2/If Action Subsystem6/If Action Subsystem6 ==
  In1 : Inport
  Action Port : ActionPort  ActionPortLabel=elseif( u1 >= 1.545)
  LUT 1.55RR : Lookup_n-D  NumberOfTableDimensions=1  BreakpointsForDimension1=[407.1524;544.2329;638.204;731.5209;824.3716;916.9086;1009.231;1101.402;1193.465;1285.447;1377.369;1469.245;1561.084;1652.895;1744.683;1836.452;1928.206]  Table=[400;500;600;700;800;900;1000;1100;1200;1300;1400;1500;1600;1700;1800;1900;2000]  InternalRulePriority=Speed  RndMeth=Simplest
  Out1 : Outport
  wires:
  In1/1 -> LUT 1.55RR/1
  LUT 1.55RR/1 -> Out1/1

== system LUT_liver_pancreas_35/If Action Subsystem6/If Action Subsystem2/If Action Subsystem6/If Action Subsystem7 ==
  In1 : Inport
  Action Port : ActionPort  ActionPortLabel=elseif( u1 >= 1.565)
  LUT 1.57RR : Lookup_n-D  NumberOfTableDimensions=1  BreakpointsForDimension1=[406.9984;543.9868;637.8844;731.108;823.8513;916.2707;1008.468;1100.509;1192.437;1284.283;1376.065;1467.8;1559.497;1651.164;1742.807;1834.43;1926.038]  Table=[400;500;600;700;800;900;1000;1100;1200;1300;1400;1500;1600;1700;1800;1900;2000]  InternalRulePriority=Speed  RndMeth=Simplest
  Out1 : Outport
  wires:
  In1/1 -> LUT 1.57RR/1
  LUT 1.57RR/1 -> Out1/1

== system LUT_liver_pancreas_35/If Action Subsystem6/If Action Subsystem2/If Action Subsystem6/If Action Subsystem8 ==
  In1 : Inport
  Action Port : ActionPort  ActionPortLabel=elseif(u1 >= 1.575)
  LUT 1.58RR : Lookup_n-D  NumberOfTableDimensions=1  BreakpointsForDimension1=[406.9228;543.8671;637.7294;730.908;823.5993;915.9616;1008.098;1100.076;1191.939;1283.717;1375.431;1467.097;1558.724;1650.32;1741.893;1833.445;1924.981]  Table=[400;500;600;700;800;900;1000;1100;1200;1300;1400;1500;1600;1700;1800;1900;2000]  InternalRulePriority=Speed  RndMeth=Simplest
  Out1 : Outport
  wires:
  In1/1 -> LUT 1.58RR/1
  LUT 1.58RR/1 -> Out1/1

== system LUT_liver_pancreas_35/If Action Subsystem6/If Action Subsystem2/If Action Subsystem6/If Action Subsystem9 ==
  In1 : Inport
  Action Port : ActionPort  ActionPortLabel=if(u1 >= 1.585)
  LUT 1.59RR : Lookup_n-D  NumberOfTableDimensions=1  BreakpointsForDimension1=[406.848;543.7495;637.5776;730.7123;823.3525;915.6587;1007.735;1099.651;1191.449;1283.161;1374.809;1466.406;1557.964;1649.492;1740.994;1832.476;1923.941]  Table=[400;500;600;700;800;900;1000;1100;1200;1300;1400;1500;1600;1700;1800;1900;2000]  InternalRulePriority=Speed  RndMeth=Simplest
  Out1 : Outport
  wires:
  In1/1 -> LUT 1.59RR/1
  LUT 1.59RR/1 -> Out1/1

== system LUT_liver_pancreas_35/If Action Subsystem6/If Action Subsystem2/If Action Subsystem7/If Action Subsystem1 ==
  In1 : Inport
  Action Port : ActionPort  ActionPortLabel=elseif( u1 >= 1.715)
  LUT 1.72RR : Lookup_n-D  NumberOfTableDimensions=1  BreakpointsForDimension1=[405.9489;542.3971;635.8614;728.511;820.5757;912.2404;1003.628;1094.818;1185.864;1276.805;1367.664;1458.462;1549.21;1639.92;1730.598;1821.251;1911.882]  Table=[400;500;600;700;800;900;1000;1100;1200;1300;1400;1500;1600;1700;1800;1900;2000]  InternalRulePriority=Speed  RndMeth=Simplest
  Out1 : Outport
  wires:
  In1/1 -> LUT 1.72RR/1
  LUT 1.72RR/1 -> Out1/1

== system LUT_liver_pancreas_35/If Action Subsystem6/If Action Subsystem2/If Action Subsystem7/If Action Subsystem10 ==
  In1 : Inport
  Action Port : ActionPort  ActionPortLabel=elseif( u1>= 1.705)
  LUT 1.71RR : Lookup_n-D  NumberOfTableDimensions=1  BreakpointsForDimension1=[406.0136;542.4906;635.978;728.6597;820.7634;912.4721;1003.907;1095.148;1186.247;1277.242;1368.157;1459.01;1549.816;1640.583;1731.32;1822.031;1912.722]  Table=[400;500;600;700;800;900;1000;1100;1200;1300;1400;1500;1600;1700;1800;1900;2000]  InternalRulePriority=Speed  RndMeth=Simplest
  Out1 : Outport
  wires:
  In1/1 -> LUT 1.71RR/1
  LUT 1.71RR/1 -> Out1/1

== system LUT_liver_pancreas_35/If Action Subsystem6/If Action Subsystem2/If Action Subsystem7/If Action Subsystem2 ==
  In1 : Inport
  Action Port : ActionPort  ActionPortLabel=else
  LUT 1.70RR : Lookup_n-D  NumberOfTableDimensions=1  BreakpointsForDimension1=[406.079;542.5857;636.0969;728.8116;820.955;912.7086;1004.192;1095.484;1186.637;1277.686;1368.658;1459.569;1550.432;1641.258;1732.054;1822.825;1913.575]  Table=[400;500;600;700;800;900;1000;1100;1200;1300;1400;1500;1600;1700;1800;1900;2000]  InternalRulePriority=Speed  RndMeth=Simplest
  Out1 : Outport
  wires:
  In1/1 -> LUT 1.70RR/1
  LUT 1.70RR/1 -> Out1/1

== system LUT_liver_pancreas_35/If Action Subsystem6/If Action Subsystem2/If Action Subsystem7/If Action Subsystem3 ==
  In1 : Inport
  Action Port : ActionPort  ActionPortLabel=elseif( u1 >= 1.725)
  LUT 1.73RR : Lookup_n-D  NumberOfTableDimensions=1  BreakpointsForDimension1=[405.8849;542.3052;635.7471;728.3654;820.392;912.0135;1003.354;1094.494;1185.489;1276.376;1367.181;1457.923;1548.615;1639.267;1729.888;1820.483;1911.056]  Table=[400;500;600;700;800;900;1000;1100;1200;1300;1400;1500;1600;1700;1800;1900;2000]  InternalRulePriority=Speed  RndMeth=Simplest
  Out1 : Outport
  wires:
  In1/1 -> LUT 1.73RR/1
  LUT 1.73RR/1 -> Out1/1

== system LUT_liver_pancreas_35/If Action Subsystem6/If Action Subsystem2/If Action Subsystem7/If Action Subsystem4 ==
  In1 : Inport
  Action Port : ActionPort  ActionPortLabel=elseif( u1 >= 1.735)
  LUT 1.74RR : Lookup_n-D  NumberOfTableDimensions=1  BreakpointsForDimension1=[405.8216;542.2149;635.6351;728.2229;820.2121;911.7912;1003.085;1094.177;1185.121;1275.955;1366.706;1457.393;1548.03;1638.626;1729.19;1819.727;1910.243]  Table=[400;500;600;700;800;900;1000;1100;1200;1300;1400;1500;1600;1700;1800;1900;2000]  InternalRulePriority=Speed  RndMeth=Simplest
  Out1 : Outport
  wires:
  In1/1 -> LUT 1.74RR/1
  LUT 1.74RR/1 -> Out1/1

== system LUT_liver_pancreas_35/If Action Subsystem6/If Action Subsystem2/If Action Subsystem7/If Action Subsystem5 ==
  In1 : Inport
  Action Port : ActionPort  ActionPortLabel=elseif( u1 >= 1.755)
  LUT 1.76RR : Lookup_n-D  NumberOfTableDimensions=1  BreakpointsForDimension1=[405.697;542.0387;635.4176;727.9467;819.8636;911.3602;1002.564;1093.56;1184.405;1275.136;1365.782;1456.361;1546.889;1637.375;1727.827;1818.253;1908.655]  Table=[400;500;600;700;800;900;1000;1100;1200;1300;1400;1500;1600;1700;1800;1900;2000]  InternalRulePriority=Speed  RndMeth=Simplest
  Out1 : Outport
  wires:
  In1/1 -> LUT 1.76RR/1
  LUT 1.76RR/1 -> Out1/1

== system LUT_liver_pancreas_35/If Action Subsystem6/If Action Subsystem2/If Action Subsystem7/If Action Subsystem6 ==
  In1 : Inport
  Action Port : ActionPort  ActionPortLabel=elseif( u1 >= 1.745)
  LUT 1.75RR : Lookup_n-D  NumberOfTableDimensions=1  BreakpointsForDimension1=[405.759;542.126;635.5253;728.0833;820.036;911.5735;1002.822;1093.866;1184.759;1275.542;1366.24;1456.873;1547.454;1637.995;1728.503;1818.984;1909.443]  Table=[400;500;600;700;800;900;1000;1100;1200;1300;1400;1500;1600;1700;1800;1900;2000]  InternalRulePriority=Speed  RndMeth=Simplest
  Out1 : Outport
  wires:
  In1/1 -> LUT 1.75RR/1
  LUT 1.75RR/1 -> Out1/1

== system LUT_liver_pancreas_35/If Action Subsystem6/If Action Subsystem2/If Action Subsystem7/If Action Subsystem7 ==
  In1 : Inport
  Action Port : ActionPort  ActionPortLabel=elseif( u1 >= 1.765)
  LUT 1.77RR : Lookup_n-D  NumberOfTableDimensions=1  BreakpointsForDimension1=[405.6357;541.9528;635.3121;727.8129;819.6948;911.1514;1002.312;1093.261;1184.056;1274.737;1365.332;1455.858;1546.332;1636.764;1727.162;1817.533;1907.88]  Table=[400;500;600;700;800;900;1000;1100;1200;1300;1400;1500;1600;1700;1800;1900;2000]  InternalRulePriority=Speed  RndMeth=Simplest
  Out1 : Outport
  wires:
  In1/1 -> LUT 1.77RR/1
  LUT 1.77RR/1 -> Out1/1

== system LUT_liver_pancreas_35/If Action Subsystem6/If Action Subsystem2/If Action Subsystem7/If Action Subsystem8 ==
  In1 : Inport
  Action Port : ActionPort  ActionPortLabel=elseif(u1 >= 1.775)
  LUT 1.78RR : Lookup_n-D  NumberOfTableDimensions=1  BreakpointsForDimension1=[405.575;541.8684;635.2087;727.6819;819.5295;910.9468;1002.064;1092.967;1183.715;1274.346;1364.889;1455.364;1545.786;1636.164;1726.509;1816.825;1907.117]  Table=[400;500;600;700;800;900;1000;1100;1200;1300;1400;1500;1600;1700;1800;1900;2000]  InternalRulePriority=Speed  RndMeth=Simplest
  Out1 : Outport
  wires:
  In1/1 -> LUT 1.78RR/1
  LUT 1.78RR/1 -> Out1/1

== system LUT_liver_pancreas_35/If Action Subsystem6/If Action Subsystem2/If Action Subsystem7/If Action Subsystem9 ==
  In1 : Inport
  Action Port : ActionPort  ActionPortLabel=if(u1 >= 1.785)
  LUT 1.79RR : Lookup_n-D  NumberOfTableDimensions=1  BreakpointsForDimension1=[405.515;541.7853;635.1074;727.5537;819.3678;910.7464;1001.821;1092.679;1183.38;1273.962;1364.455;1454.879;1545.248;1635.574;1725.865;1816.128;1906.367]  Table=[400;500;600;700;800;900;1000;1100;1200;1300;1400;1500;1600;1700;1800;1900;2000]  InternalRulePriority=Speed  RndMeth=Simplest
  Out1 : Outport
  wires:
  In1/1 -> LUT 1.79RR/1
  LUT 1.79RR/1 -> Out1/1

== system LUT_liver_pancreas_35/If Action Subsystem6/If Action Subsystem2/If Action Subsystem8/If Action Subsystem1 ==
  In1 : Inport
  Action Port : ActionPort  ActionPortLabel=elseif( u1 >= 1.815)
  LUT 1.82RR : Lookup_n-D  NumberOfTableDimensions=1  BreakpointsForDimension1=[405.3385;541.5443;634.8151;727.185;818.9026;910.1697;1001.122;1091.849;1182.411;1272.851;1363.198;1453.472;1543.689;1633.862;1723.997;1814.103;1904.184]  Table=[400;500;600;700;800;900;1000;1100;1200;1300;1400;1500;1600;1700;1800;1900;2000]  InternalRulePriority=Speed  RndMeth=Simplest
  Out1 : Outport
  wires:
  In1/1 -> LUT 1.82RR/1
  LUT 1.82RR/1 -> Out1/1

== system LUT_liver_pancreas_35/If Action Subsystem6/If Action Subsystem2/If Action Subsystem8/If Action Subsystem10 ==
  In1 : Inport
  Action Port : ActionPort  ActionPortLabel=elseif( u1>= 1.805)
  LUT 1.81RR : Lookup_n-D  NumberOfTableDimensions=1  BreakpointsForDimension1=[405.3967;541.6233;634.9106;727.3053;819.0544;910.3579;1001.35;1092.12;1182.728;1273.215;1363.609;1453.933;1544.2;1634.423;1724.61;1814.767;1904.9]  Table=[400;500;600;700;800;900;1000;1100;1200;1300;1400;1500;1600;1700;1800;1900;2000]  InternalRulePriority=Speed  RndMeth=Simplest
  Out1 : Outport
  wires:
  In1/1 -> LUT 1.81RR/1
  LUT 1.81RR/1 -> Out1/1

== system LUT_liver_pancreas_35/If Action Subsystem6/If Action Subsystem2/If Action Subsystem8/If Action Subsystem2 ==
  In1 : Inport
  Action Port : ActionPort  ActionPortLabel=else
  LUT 1.80RR : Lookup_n-D  NumberOfTableDimensions=1  BreakpointsForDimension1=[405.4556;541.7036;635.008;727.4282;819.2094;910.5501;1001.583;1092.397;1183.051;1273.585;1364.028;1454.402;1544.72;1634.994;1725.232;1815.442;1905.628]  Table=[400;500;600;700;800;900;1000;1100;1200;1300;1400;1500;1600;1700;1800;1900;2000]  InternalRulePriority=Speed  RndMeth=Simplest
  Out1 : Outport
  wires:
  In1/1 -> LUT 1.80RR/1
  LUT 1.80RR/1 -> Out1/1

== system LUT_liver_pancreas_35/If Action Subsystem6/If Action Subsystem2/If Action Subsystem8/If Action Subsystem3 ==
  In1 : Inport
  Action Port : ActionPort  ActionPortLabel=elseif( u1 >= 1.825)
  LUT 1.83RR : Lookup_n-D  NumberOfTableDimensions=1  BreakpointsForDimension1=[405.2809;541.4665;634.7215;727.0672;818.7541;909.9853;1000.898;1091.582;1182.1;1272.494;1362.793;1453.019;1543.187;1633.309;1723.394;1813.449;1903.479]  Table=[400;500;600;700;800;900;1000;1100;1200;1300;1400;1500;1600;1700;1800;1900;2000]  InternalRulePriority=Speed  RndMeth=Simplest
  Out1 : Outport
  wires:
  In1/1 -> LUT 1.83RR/1
  LUT 1.83RR/1 -> Out1/1

== system LUT_liver_pancreas_35/If Action Subsystem6/If Action Subsystem2/If Action Subsystem8/If Action Subsystem4 ==
  In1 : Inport
  Action Port : ActionPort  ActionPortLabel=elseif( u1 >= 1.835)
  LUT 1.84RR : Lookup_n-D  NumberOfTableDimensions=1  BreakpointsForDimension1=[405.2239;541.39;634.6297;726.952;818.6087;909.8048;1000.678;1091.321;1181.795;1272.143;1362.396;1452.574;1542.693;1632.766;1722.801;1812.806;1902.785]  Table=[400;500;600;700;800;900;1000;1100;1200;1300;1400;1500;1600;1700;1800;1900;2000]  InternalRulePriority=Speed  RndMeth=Simplest
  Out1 : Outport
  wires:
  In1/1 -> LUT 1.84RR/1
  LUT 1.84RR/1 -> Out1/1

== system LUT_liver_pancreas_35/If Action Subsystem6/If Action Subsystem2/If Action Subsystem8/If Action Subsystem5 ==
  In1 : Inport
  Action Port : ActionPort  ActionPortLabel=elseif( u1 >= 1.855)
  LUT 1.86RR : Lookup_n-D  NumberOfTableDimensions=1  BreakpointsForDimension1=[405.1115;541.2407;634.4515;726.7287;818.3271;909.455;1000.253;1090.814;1181.202;1271.461;1361.622;1451.706;1541.73;1631.706;1721.644;1811.55;1901.429]  Table=[400;500;600;700;800;900;1000;1100;1200;1300;1400;1500;1600;1700;1800;1900;2000]  InternalRulePriority=Speed  RndMeth=Simplest
  Out1 : Outport
  wires:
  In1/1 -> LUT 1.86RR/1
  LUT 1.86RR/1 -> Out1/1

== system LUT_liver_pancreas_35/If Action Subsystem6/If Action Subsystem2/If Action Subsystem8/If Action Subsystem6 ==
  In1 : Inport
  Action Port : ActionPort  ActionPortLabel=elseif( u1 >= 1.845)
  LUT 1.85RR : Lookup_n-D  NumberOfTableDimensions=1  BreakpointsForDimension1=[405.1674;541.3148;634.5397;726.8391;818.4664;909.6281;1000.463;1091.065;1181.496;1271.799;1362.005;1452.136;1542.208;1632.232;1722.218;1812.173;1902.102]  Table=[400;500;600;700;800;900;1000;1100;1200;1300;1400;1500;1600;1700;1800;1900;2000]  InternalRulePriority=Speed  RndMeth=Simplest
  Out1 : Outport
  wires:
  In1/1 -> LUT 1.85RR/1
  LUT 1.85RR/1 -> Out1/1

== system LUT_liver_pancreas_35/If Action Subsystem6/If Action Subsystem2/If Action Subsystem8/If Action Subsystem7 ==
  In1 : Inport
  Action Port : ActionPort  ActionPortLabel=elseif( u1 >= 1.865)
  LUT 1.87RR : Lookup_n-D  NumberOfTableDimensions=1  BreakpointsForDimension1=[405.0562;541.1679;634.3651;726.6205;818.1908;909.2855;1000.046;1090.568;1180.914;1271.13;1361.245;1451.283;1541.261;1631.19;1721.079;1810.936;1900.767]  Table=[400;500;600;700;800;900;1000;1100;1200;1300;1400;1500;1600;1700;1800;1900;2000]  InternalRulePriority=Speed  RndMeth=Simplest
  Out1 : Outport
  wires:
  In1/1 -> LUT 1.87RR/1
  LUT 1.87RR/1 -> Out1/1

== system LUT_liver_pancreas_35/If Action Subsystem6/If Action Subsystem2/If Action Subsystem8/If Action Subsystem8 ==
  In1 : Inport
  Action Port : ActionPort  ActionPortLabel=elseif(u1 >= 1.875)
  LUT 1.88RR : Lookup_n-D  NumberOfTableDimensions=1  BreakpointsForDimension1=[405.0014;541.0962;634.2803;726.5147;818.0575;909.1196;999.8442;1090.327;1180.632;1270.804;1360.875;1450.868;1540.799;1630.681;1720.523;1810.333;1900.115]  Table=[400;500;600;700;800;900;1000;1100;1200;1300;1400;1500;1600;1700;1800;1900;2000]  InternalRulePriority=Speed  RndMeth=Simplest
  Out1 : Outport
  wires:
  In1/1 -> LUT 1.88RR/1
  LUT 1.88RR/1 -> Out1/1

== system LUT_liver_pancreas_35/If Action Subsystem6/If Action Subsystem2/If Action Subsystem8/If Action Subsystem9 ==
  In1 : Inport
  Action Port : ActionPort  ActionPortLabel=if(u1 >= 1.885)
  LUT 1.89RR : Lookup_n-D  NumberOfTableDimensions=1  BreakpointsForDimension1=[404.9471;541.0256;634.1972;726.4111;817.9269;908.9572;999.646;1090.09;1180.354;1270.484;1360.512;1450.46;1540.345;1630.181;1719.976;1809.738;1899.473]  Table=[400;500;600;700;800;900;1000;1100;1200;1300;1400;1500;1600;1700;1800;1900;2000]  InternalRulePriority=Speed  RndMeth=Simplest
  Out1 : Outport
  wires:
  In1/1 -> LUT 1.89RR/1
  LUT 1.89RR/1 -> Out1/1
